simulink model "SinCos"  (R2020b)
settings: Solver=VariableStepAuto  StartTime=0.0  StopTime=25  RelTol=1e-3
settings Model: Creator=riwakaram  LastModifiedBy=riwakaram

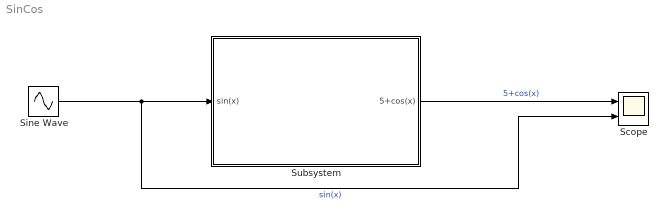
== system SinCos ==
  Scope : Scope  NumInputPorts=2
  Sine Wave : Sin  SampleTime=0
  Subsystem : Subsystem
  wires:
  Sine Wave/1 -> Scope/2, Subsystem/1(sin(x))  "sin(x)"
  Subsystem/1(5+cos(x)) -> Scope/1  "5+cos(x)"

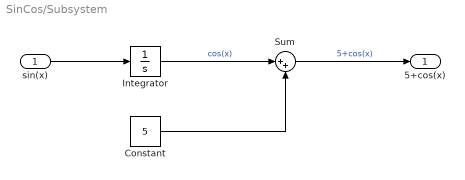
== system SinCos/Subsystem ==
  sin(x) : Inport
  Constant : Constant  Value=5
  Integrator : Integrator
  Sum : Sum  Inputs=|++
  5+cos(x) : Outport
  wires:
  Sum/1 -> 5+cos(x)/1  "5+cos(x)"
  sin(x)/1 -> Integrator/1
  Constant/1 -> Sum/2
  Integrator/1 -> Sum/1  "cos(x)"
